simulink model "Work1"  (R2015b)
settings: Solver=FixedStepAuto  StartTime=0.0  StopTime=21  FixedStep=1  RelTol=1e-3
settings Model: Creator=User  LastModifiedBy=Druzhinin_Vasily

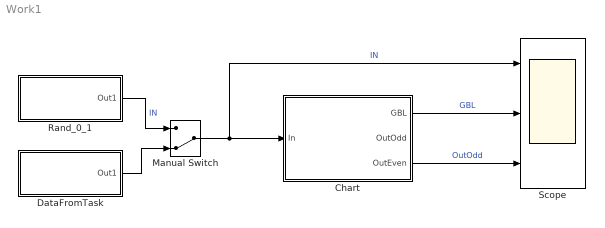
== system Work1 ==
  Chart : Stateflow chart  TreatAsAtomicUnit=on
  DataFromTask : Subsystem
  Manual Switch : ManualSwitch  CurrentSetting=0
  Rand_0_1 : Subsystem
  Scope : Scope  NumInputPorts=3
  wires:
  Manual Switch/1 -> Scope/1, Chart/1(In)  "IN"
  Chart/1(GBL) -> Scope/2  "GBL"
  Chart/3(OutEven) -> Scope/3  "OutOdd"
  DataFromTask/1(Out1) -> Manual Switch/2
  Rand_0_1/1(Out1) -> Manual Switch/1  "IN"

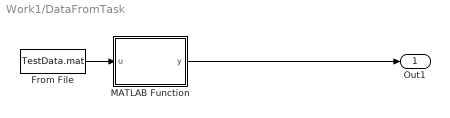
== system Work1/DataFromTask ==
  From File : FromFile  FileName=TestData.mat  SampleTime=1
  MATLAB Function : MATLAB Function  TreatAsAtomicUnit=on
  Out1 : Outport
  wires:
  MATLAB Function/1(y) -> Out1/1
  From File/1 -> MATLAB Function/1(u)

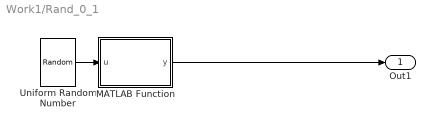
== system Work1/Rand_0_1 ==
  MATLAB Function : MATLAB Function  TreatAsAtomicUnit=on
  Uniform Random Number : UniformRandomNumber  Minimum=0  SampleTime=1
  Out1 : Outport
  wires:
  Uniform Random Number/1 -> MATLAB Function/1(u)
  MATLAB Function/1(y) -> Out1/1

== matlab function Work1/DataFromTask/MATLAB Function ==
  data: u input; y output
function y = fcn(u)
%#codegen
if u >= 0.5
    y=true;
else
    y=false;
end;

== matlab function Work1/Rand_0_1/MATLAB Function ==
  data: u input; y output
function y = fcn(u)
%#codegen
if u >= 0.5
    y=true;
else
    y=false;
end;

== stateflow chart Work1/Chart ==
  state StartMessage
    entry:
    GBL = GBL + 1;
  state StopMessage
    entry:
    GBL = GBL;
  state StopMessage1
    entry:
    if (rem(GBL,2)==0 && GBL~=0)
    OutEven=true;
    else
    OutEven = false;
    end;
    OutOdd=rem(GBL,2)
    GBL = 0;
  (default) -> (junction 15)
  StartMessage -> (junction 15)
  StopMessage1 -> (junction 15)
  (junction 15) -> StartMessage [order 2] : [In==1]
  (junction 15) -> StopMessage [order 1] : [In == 0]
  StopMessage -> StartMessage [order 2] : [In==1]
  StopMessage -> StopMessage1 [order 1] : [In==0]
  data: In input boolean; GBL output =0; OutOdd output; OutEven output boolean
